simulink model "scen2"  (R2023b)
settings: Solver=VariableStepAuto  StartTime=0.0  StopTime=50  RelTol=1e-3
libraries: slpidlib x2, simulink_extras x1, simulink x1, SignalEditorBlockLib x1
settings Model: Creator=yusufcagriogut  LastModifiedBy=yusufcagriogut

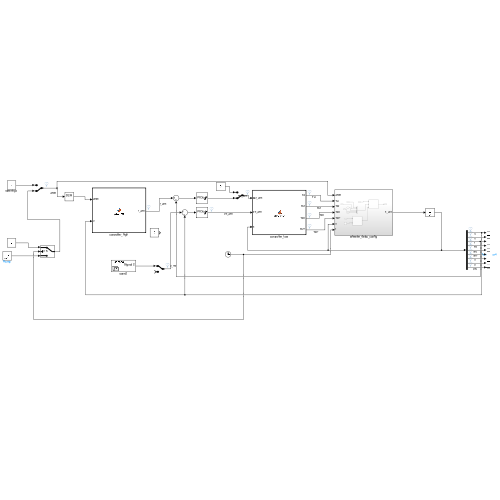
[thumbnail: Simulink's stored preview of the top-level diagram]
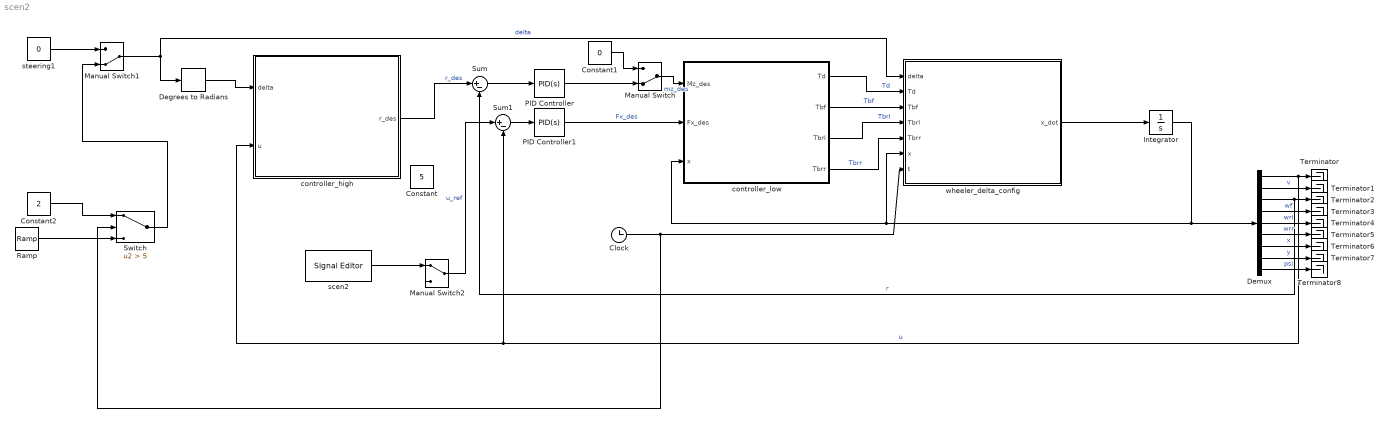
== system scen2 ==
  Clock : Clock
  Constant : Constant  Value=5
  Constant1 : Constant  Value=0
  Constant2 : Constant  Value=2
  Degrees to Radians : simulink_extras/Transformations/Degrees to Radians
  Demux : Demux  Outputs=9
  Integrator : Integrator  InitialCondition=[25; 0; 0; 25/0.28; 25/0.28; 25/0.28; 0; 0; 0]
  Manual Switch : ManualSwitch  CurrentSetting=0
  Manual Switch1 : ManualSwitch  CurrentSetting=0
  Manual Switch2 : ManualSwitch
  PID Controller : slpidlib/PID Controller  Controller=PID  Form=Parallel  TimeDomain=Continuous-time  UseExternalTs=off  SampleTime=-1  IntegratorMethod=Forward Euler  FilterMethod=Forward Euler  ControllerParametersSource=internal  P=1500  I=500  UseKiTs=off  D=0  N=100  UseFilter=on  TunerSelectOption=Transfer Function Based (PID Tuner App)  InitialConditionSource=internal  InitialConditionForIntegrator=0  InitialConditionForFilter=0  DifferentiatorICPrevScaledInput=0  ExternalReset=none  TrackingMode=off  Kt=1  LimitOutput=on  SatLimitsSource=internal  UpperSaturationLimit=250  LowerSaturationLimit=-250  LinearizeAsGain=on  AntiWindupMode=clamping  Kb=1  LimitIntegrator=off  UpperIntegratorSaturationLimit=inf  LowerIntegratorSaturationLimit=-inf  POutMin=[]  POutMax=[]  IOutMin=[]  IOutMax=[]  DOutMin=[]  DOutMax=[]  NOutMin=[]  NOutMax=[]  SumOutMin=[]  SumOutMax=[]  SaturationOutMin=[]  SaturationOutMax=[]  PParamMin=[]  PParamMax=[]  IParamMin=[]  IParamMax=[]  DParamMin=[]  DParamMax=[]  NParamMin=[]  NParamMax=[]  KbParamMin=[]  KbParamMax=[]  KtParamMin=[]  KtParamMax=[]  KbOutMin=[]  KbOutMax=[]  KtOutMin=[]  KtOutMax=[]  IntegratorOutMin=[]  IntegratorOutMax=[]  FilterOutMin=[]  FilterOutMax=[]  SumI1OutMin=[]  SumI1OutMax=[]  SumI2OutMin=[]  SumI2OutMax=[]  SumI3OutMin=[]  SumI3OutMax=[]  SumI4OutMin=[]  SumI4OutMax=[]  SumDOutMin=[]  SumDOutMax=[]  DifferentiatorOutMin=[]  DifferentiatorOutMax=[]  FilterDiffOutCoefMin=[]  FilterDiffOutCoefMax=[]  ReciprocalOutMin=[]  ReciprocalOutMax=[]  SumDenOutMin=[]  SumDenOutMax=[]  SumNumOutMin=[]  SumNumOutMax=[]  DivideOutMin=[]  DivideOutMax=[]  UdiffTsProdOutMin=[]  UdiffTsProdOutMax=[]  NTsProdOutMin=[]  NTsProdOutMax=[]  UintegralTsProdOutMin=[]  UintegralTsProdOutMax=[]  UngainTsProdOutMin=[]  UngainTsProdOutMax=[]  ClampingZeroOutDataTypeStr=Inherit: Inherit via back propagation  ClampingZeroOutMin=[]  ClampingZeroOutMax=[]  FilterDenConstantOutDataTypeStr=Inherit: Inherit via back propagation  FilterDenConstantOutMin=[]  FilterDenConstantOutMax=[]  PCopyOutDataTypeStr=Inherit: Inherit via back propagation  PCopyOutMin=[]  PCopyOutMax=[]  NCopyOutDataTypeStr=Inherit: Inherit via back propagation  NCopyOutMin=[]  NCopyOutMax=[]  IntegratorContinuousStateAttributes=''  IntegratorStateMustResolveToSignalObject=off  IntegratorRTWStateStorageClass=Auto  FilterContinuousStateAttributes=''  FilterStateMustResolveToSignalObject=off  FilterRTWStateStorageClass=Auto  ParallelPVariant=InternalParameters  IdealPVariant=Disabled  IVariant=InternalParameters  DVariant=InternalParameters  IntegratorVariant=Continuous  SatVariant=Enabled  AWVariant=ContClampingParallel  PCopyVariant=Disabled  TRVariant=Disabled  FdbkBlocksVariant=Forward  IdealPFdbkVariant=Disabled  SatFdbkVariant=Disabled  DerivativeFilterVariant=ContFilter  NVariant=InternalParameters  NCopyVariant=Disabled  FilterICVariant=InternalICsFilter  IntegratorICVariant=InternalICs  ExternalResetVariant=Disabled  TRSumVariant=Passthrough  SumFdbkVariant=Disabled  SumVariant=Sum_PID  TsampFilterVariant=InternalTs  TsampNgainVariant=Passthrough  TsampIntegralVariant=Disabled_SignalSpec  ExternalSaturationOutDataTypeStr=Inherit: Same as second input
  PID Controller1 : slpidlib/PID Controller  Controller=PID  Form=Parallel  TimeDomain=Continuous-time  UseExternalTs=off  SampleTime=-1  IntegratorMethod=Forward Euler  FilterMethod=Forward Euler  ControllerParametersSource=internal  P=800  I=200  UseKiTs=off  D=0  N=100  UseFilter=on  TunerSelectOption=Transfer Function Based (PID Tuner App)  InitialConditionSource=internal  InitialConditionForIntegrator=0  InitialConditionForFilter=0  DifferentiatorICPrevScaledInput=0  ExternalReset=none  TrackingMode=off  Kt=1  LimitOutput=on  SatLimitsSource=internal  UpperSaturationLimit=1430  LowerSaturationLimit=-6000  LinearizeAsGain=on  AntiWindupMode=clamping  Kb=1  LimitIntegrator=off  UpperIntegratorSaturationLimit=inf  LowerIntegratorSaturationLimit=-inf  POutMin=[]  POutMax=[]  IOutMin=[]  IOutMax=[]  DOutMin=[]  DOutMax=[]  NOutMin=[]  NOutMax=[]  SumOutMin=[]  SumOutMax=[]  SaturationOutMin=[]  SaturationOutMax=[]  PParamMin=[]  PParamMax=[]  IParamMin=[]  IParamMax=[]  DParamMin=[]  DParamMax=[]  NParamMin=[]  NParamMax=[]  KbParamMin=[]  KbParamMax=[]  KtParamMin=[]  KtParamMax=[]  KbOutMin=[]  KbOutMax=[]  KtOutMin=[]  KtOutMax=[]  IntegratorOutMin=[]  IntegratorOutMax=[]  FilterOutMin=[]  FilterOutMax=[]  SumI1OutMin=[]  SumI1OutMax=[]  SumI2OutMin=[]  SumI2OutMax=[]  SumI3OutMin=[]  SumI3OutMax=[]  SumI4OutMin=[]  SumI4OutMax=[]  SumDOutMin=[]  SumDOutMax=[]  DifferentiatorOutMin=[]  DifferentiatorOutMax=[]  FilterDiffOutCoefMin=[]  FilterDiffOutCoefMax=[]  ReciprocalOutMin=[]  ReciprocalOutMax=[]  SumDenOutMin=[]  SumDenOutMax=[]  SumNumOutMin=[]  SumNumOutMax=[]  DivideOutMin=[]  DivideOutMax=[]  UdiffTsProdOutMin=[]  UdiffTsProdOutMax=[]  NTsProdOutMin=[]  NTsProdOutMax=[]  UintegralTsProdOutMin=[]  UintegralTsProdOutMax=[]  UngainTsProdOutMin=[]  UngainTsProdOutMax=[]  ClampingZeroOutDataTypeStr=Inherit: Inherit via back propagation  ClampingZeroOutMin=[]  ClampingZeroOutMax=[]  FilterDenConstantOutDataTypeStr=Inherit: Inherit via back propagation  FilterDenConstantOutMin=[]  FilterDenConstantOutMax=[]  PCopyOutDataTypeStr=Inherit: Inherit via back propagation  PCopyOutMin=[]  PCopyOutMax=[]  NCopyOutDataTypeStr=Inherit: Inherit via back propagation  NCopyOutMin=[]  NCopyOutMax=[]  IntegratorContinuousStateAttributes=''  IntegratorStateMustResolveToSignalObject=off  IntegratorRTWStateStorageClass=Auto  FilterContinuousStateAttributes=''  FilterStateMustResolveToSignalObject=off  FilterRTWStateStorageClass=Auto  ParallelPVariant=InternalParameters  IdealPVariant=Disabled  IVariant=InternalParameters  DVariant=InternalParameters  IntegratorVariant=Continuous  SatVariant=Enabled  AWVariant=ContClampingParallel  PCopyVariant=Disabled  TRVariant=Disabled  FdbkBlocksVariant=Forward  IdealPFdbkVariant=Disabled  SatFdbkVariant=Disabled  DerivativeFilterVariant=ContFilter  NVariant=InternalParameters  NCopyVariant=Disabled  FilterICVariant=InternalICsFilter  IntegratorICVariant=InternalICs  ExternalResetVariant=Disabled  TRSumVariant=Passthrough  SumFdbkVariant=Disabled  SumVariant=Sum_PID  TsampFilterVariant=InternalTs  TsampNgainVariant=Passthrough  TsampIntegralVariant=Disabled_SignalSpec  ExternalSaturationOutDataTypeStr=Inherit: Same as second input
  Ramp : simulink/Sources/Ramp  slope=2/5  start=0  InitialOutput=0
  Sum : Sum  Inputs=|+-
  Sum1 : Sum  Inputs=|+-
  Switch : Switch  Criteria=u2 > Threshold  Threshold=5  SaturateOnIntegerOverflow=off  InputSameDT=off
  Terminator{,1..8} (9 alike) : Terminator
  controller_high : MATLAB Function  TreatAsAtomicUnit=on
  controller_low : MATLAB Function  TreatAsAtomicUnit=on
  scen2 : SignalEditorBlockLib/Signal Editor  FileName=sig1.mat  ActiveScenario=Scenario  ActiveSignal=Signal 2  IsBus=off  OutputBusObjectStr=Bus: BusObject  SampleTime=0  Interpolate=off  ZeroCross=off  OutputAfterFinalValue=Setting to zero  Unit=inherit  PreserveSignalName=on  ApplySigPropsToAllScenarios=on  ApplySigPropsToAllSignals=off
  steering1 : Constant  Value=0
  wheeler_delta_config : Subsystem
  wires:
  wheeler_delta_config/1(x_dot) -> Integrator/1
  Integrator/1 -> wheeler_delta_config/6(x), controller_low/3(x), Demux/1
  Demux/1 -> Sum1/2, controller_high/2(u), Terminator/1  "u"
  Demux/2 -> Terminator1/1  "v"
  Demux/3 -> Sum/2, Terminator2/1  "r"
  Demux/4 -> Terminator3/1  "wf"
  Demux/5 -> Terminator4/1  "wrl"
  Demux/6 -> Terminator5/1  "wrr"
  Demux/7 -> Terminator6/1  "x"
  Demux/8 -> Terminator7/1  "y"
  Demux/9 -> Terminator8/1  "psi"
  Manual Switch1/1 -> Degrees to Radians/1, wheeler_delta_config/1(delta)  "delta"
  Degrees to Radians/1 -> controller_high/1(delta)
  controller_low/1(Td) -> wheeler_delta_config/2(Td)  "Td"
  controller_low/2(Tbf) -> wheeler_delta_config/3(Tbf)  "Tbf"
  controller_low/3(Tbrl) -> wheeler_delta_config/4(Tbrl)  "Tbrl"
  controller_low/4(Tbrr) -> wheeler_delta_config/5(Tbrr)  "Tbrr"
  PID Controller/1 -> Manual Switch/2
  Sum/1 -> PID Controller/1
  controller_high/1(r_des) -> Sum/1  "r_des"
  PID Controller1/1 -> controller_low/2(Fx_des)  "Fx_des"
  Sum1/1 -> PID Controller1/1
  Manual Switch2/1 -> Sum1/1  "u_ref"
  Clock/1 -> Switch/2, wheeler_delta_config/7(t)
  Constant1/1 -> Manual Switch/1
  Manual Switch/1 -> controller_low/1(Mz_des)  "mz_des"
  steering1/1 -> Manual Switch1/1
  scen2/1 -> Manual Switch2/1
  Ramp/1 -> Switch/3
  Constant2/1 -> Switch/1
  Switch/1 -> Manual Switch1/2

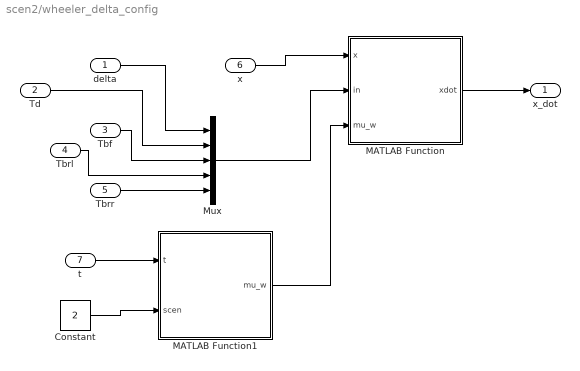
== system scen2/wheeler_delta_config ==
  delta : Inport
  Td : Inport  Port=2
  Tbf : Inport  Port=3
  Tbrl : Inport  Port=4
  Tbrr : Inport  Port=5
  x : Inport  Port=6  PortDimensions=[9,1]
  t : Inport  Port=7
  Constant : Constant  Value=2
  MATLAB Function : MATLAB Function  TreatAsAtomicUnit=on
  MATLAB Function1 : MATLAB Function  TreatAsAtomicUnit=on
  Mux : Mux  Inputs=5
  x_dot : Outport  PortDimensions=[9,1]
  wires:
  MATLAB Function/1(xdot) -> x_dot/1
  x/1 -> MATLAB Function/1(x)
  delta/1 -> Mux/1
  Td/1 -> Mux/2
  Tbf/1 -> Mux/3
  Tbrl/1 -> Mux/4
  Tbrr/1 -> Mux/5
  Mux/1 -> MATLAB Function/2(in)
  MATLAB Function1/1(mu_w) -> MATLAB Function/3(mu_w)
  t/1 -> MATLAB Function1/1(t)
  Constant/1 -> MATLAB Function1/2(scen)

== matlab function scen2/controller_low ==
  data: Mz_des input; Td output; Fx_des input; x input; Tbf output; Tbrl output; Tbrr output
function [Td, Tbf, Tbrl, Tbrr] = allocator(Mz_des, Fx_des, x)
%#codegen
Re=0.28; tr=0.60; Tb_max=1200; Td_max=400;
mu=0.90; g=9.81; m=500; lf=0.85; L=1.60;
Fzr = m*g*lf/(2*L);
Tb_grip = mu*Fzr*Re;

% required brake-torque difference to make Mz_des
dT = (Re/tr) * Mz_des;          % positive dT brakes rear-left more

% baseline longitudinal brake demand (only when decelerating)
if Fx_des >= 0
    Td = min(Fx_des*Re, Td_max);
    Tb_base = 0;
else
    Td = 0;
    Tb_base = min(-Fx_des*Re, Tb_max);
end

% IMPORTANT: give the differential a baseline so neither side goes negative.
% Use at least half the differential magnitude as the floor.
half = 0.5*abs(dT);
base = max(Tb_base, half);       % guarantees both brakes stay >= 0

Tbrl = base + 0.5*dT;
Tbrr = base - 0.5*dT;

% if we're in pure drive (Fx_des>0) and yaw needs braking, cut drive
if Fx_des >= 0 && abs(dT) > 1e-6
    % Td = 0;                      % don't drive and brake at the same time
end

Tbf = Tb_base;                   % front brake follows longitudinal demand only

% saturate
lim = min(Tb_max, Tb_grip);
Tbrl = max(0, min(Tbrl, lim));
Tbrr = max(0, min(Tbrr, lim));
end

== matlab function scen2/wheeler_delta_config/MATLAB Function ==
  data: x input; xdot output; in input; mu_w input
function xdot = trike_plant(x, in, mu_w)
%#codegen
% 9-state nonlinear plant: front-driven, rear differential-braking delta trike.
%   x  = [u; v; r; wf; wrl; wrr; X; Y; psi]
%   in = [delta; Td; Tb_f; Tb_rl; Tb_rr]
%   xdot returned in the same order as x.

% ---------------- parameters (match trike_params.m) ----------------
g=9.81;  m=500;  Iz=550;  h=0.50;
lf=0.85; lr=0.75; L=lf+lr; tr=0.60;
Iw=1.0;  Re=0.28;
mu_f  = mu_w(1);
mu_rl = mu_w(2);
mu_rr = mu_w(3);
Calf=30000; Calr=28000; Cs=50000;
Fzf = m*g*lr/L;            % static front load
Fzr = m*g*lf/(2*L);       % static load on EACH rear wheel
rho=1.225; Cd=0.6; Af=1.8;
eps_v=0.5;                 % low-speed slip guard

% ---------------- unpack state and input ----------------
u   = x(1);  v   = x(2);  r   = x(3);
wf  = x(4);  wrl = x(5);  wrr = x(6);
psi = x(9);

delta = in(1);  Td = in(2);
Tbf = in(3);    Tbrl = in(4);  Tbrr = in(5);

% ---------------- contact-point velocities ----------------
% front (lf,0), rear-left (-lr,+tr), rear-right (-lr,-tr)
% longitudinal component of each wheel along its own heading
Vf_long  =  u*cos(delta) + (v + lf*r)*sin(delta);
Vrl_long =  u - tr*r;
Vrr_long =  u + tr*r;

% ---------------- slip angles ----------------
ux = max(u, eps_v);                 % guard division
alpha_f  = delta - atan2( (v + lf*r), ux );
alpha_rl =       - atan2( (v - lr*r), max(u - tr*r, eps_v) );
alpha_rr =       - atan2( (v - lr*r), max(u + tr*r, eps_v) );

% ---------------- slip ratios ----------------
sf  = (Re*wf  - Vf_long ) / max(max(abs(Re*wf ), abs(Vf_long )), eps_v);
srl = (Re*wrl - Vrl_long) / max(max(abs(Re*wrl), abs(Vrl_long)), eps_v);
srr = (Re*wrr - Vrr_long) / max(max(abs(Re*wrr), abs(Vrr_long)), eps_v);

% ---------------- tire forces (linear + friction-circle clamp) ----------------
% longitudinal
Fxf  = Cs*sf;
Fxrl = Cs*srl;
Fxrr = Cs*srr;
% lateral (front 1 tire, each rear 1 tire)
Fyf  = Calf*alpha_f;
Fyrl = Calr*alpha_rl;
Fyrr = Calr*alpha_rr;

% friction circle: scale each tire's force vector to mu*Fz
[Fxf , Fyf ] = clampCircle(Fxf , Fyf , mu_f*Fzf);
[Fxrl, Fyrl] = clampCircle(Fxrl, Fyrl, mu_rl*Fzr);
[Fxrr, Fyrr] = clampCircle(Fxrr, Fyrr, mu_rr*Fzr);

% ---------------- resolve into body frame ----------------
Fx_f =  Fxf*cos(delta) - Fyf*sin(delta);
Fy_f =  Fxf*sin(delta) + Fyf*cos(delta);

Faero = 0.5*rho*Cd*Af*u*abs(u);

sumFx = Fx_f + Fxrl + Fxrr - Faero;
sumFy = Fy_f + Fyrl + Fyrr;

% yaw moment about CG  (note the differential-braking term)
Mz =  lf*(Fxf*sin(delta) + Fyf*cos(delta)) ...
    - lr*(Fyrl + Fyrr) ...
    + tr*(Fxrr - Fxrl);

% ---------------- rigid-body accelerations ----------------
udot = sumFx/m + v*r;
vdot = sumFy/m - u*r;
rdot = Mz/Iz;

% ---------------- wheel-spin dynamics ----------------
wfdot  = ( Td - Tbf  - Re*Fxf  ) / Iw;
wrldot = (    - Tbrl - Re*Fxrl ) / Iw;
wrrdot = (    - Tbrr - Re*Fxrr ) / Iw;

% ---------------- global pose ----------------
Xdot   = u*cos(psi) - v*sin(psi);
Ydot   = u*sin(psi) + v*cos(psi);
psidot = r;

% ---------------- assemble ----------------
xdot = [udot; vdot; rdot; wfdot; wrldot; wrrdot; Xdot; Ydot; psidot];
end

% ===================================================================
function [Fx, Fy] = clampCircle(Fx, Fy, Fmax)
% scale (Fx,Fy) down so its magnitude never exceeds Fmax
Fmag = sqrt(Fx^2 + Fy^2);
if Fmag > Fmax && Fmag > 0
    sc = Fmax / Fmag;
    Fx = Fx*sc;
    Fy = Fy*sc;
end
end

== matlab function scen2/controller_high ==
  data: delta input; r_des output; u input
function r_des = yaw_ref(delta, u)
%#codegen
% Desired yaw rate from a steady-state bicycle model, saturated by grip.
L   = 1.60;        % wheelbase (lf+lr)
Kus = 0.0015;      % understeer gradient [rad/(m/s^2)]  [TUNE]
mu  = 0.90; g = 9.81;
uu  = max(u, 0.5);

r_lin = delta * uu / (L + Kus*uu^2);   % linear target
r_max = mu*g / uu;                      % grip ceiling |ay|<=mu*g
r_des = max(min(r_lin, r_max), -r_max);

== matlab function scen2/wheeler_delta_config/MATLAB Function1 ==
  data: t input; mu_w output; scen input
function mu_w = road_splitmu(t, scen)
%#codegen
% Split-mu surface: LEFT side high grip, RIGHT side ice, from t=10s on.
% mu_w = [mu_front; mu_rear_left; mu_rear_right]
if scen==1
    mu_hi = 0.90;
    mu_lo = 0.30;
elseif scen==2
    mu_hi = 0.60;
    mu_lo = 0.60;
else
    mu_hi = 0.60;
    mu_lo = 0.60;
end


if t < 10
    mu_w = [mu_hi; mu_hi; mu_hi];     % uniform dry road before the event
else
    mu_w = [mu_hi; mu_hi; mu_lo];     % right rear hits ice
end
